simulink model "Motor_Cmd_varY"  (Simulink 7.9)
settings: Solver=FixedStepDiscrete  StartTime=0.0  StopTime=10  RelTol=1e-3  SampleTimeConstraint=STIndependent
PreLoadFcn:
  | Motor_Cmd_varY_selfinit
values from neighbouring files (symbols this model uses):
  lockDoor_cmdMotorVoltageValue = mpt.Parameter    [Motor_Cmd_varY_selfinit.m]
libraries: simulink x1
settings Model: RequirementInfo="{}  %GIDa_76f203d0_57c5_4172_aee2_9207869380ab"  Creator=fguerin  LastModifiedBy=klindqvi  CovMetricSettings=dc  CovHTMLOptions=-aTS=1 -bRG=1 -bTC=1 -hTR=0 -nFC=0 -scm=1 -bcm=1 -xEv=0  CovModelRefEnable=all
settings DataIOCC: ExternalInput=[t,u]  LimitDataPoints=off  SaveOutput=off  DSMLogging=off  SaveTime=off  SignalLoggingName=logsOut
settings OptimizationCC: InlineParams=on  InlineInvariantSignals=on  EnhancedBackFolding=on  ZeroExternalMemoryAtStartup=off  ZeroInternalMemoryAtStartup=off  EfficientFloat2IntCast=on  OptimizeModelRefInitCode=on  LifeSpan=1
settings DebuggingCC: ReadBeforeWriteMsg=EnableAllAsError  WriteAfterWriteMsg=EnableAllAsError  WriteAfterReadMsg=EnableAllAsError  AlgebraicLoopMsg=error  ArtificialAlgebraicLoopMsg=error  SaveWithDisabledLinksMsg=error  SaveWithParameterizedLinksMsg=error  CheckExecutionContextPreStartOutputMsg=on  CheckExecutionContextRuntimeOutputMsg=on  BlockPriorityViolationMsg=error  SolverPrmCheckMsg=none  MultiTaskCondExecSysMsg=warning  MultiTaskRateTransMsg=warning  IntegerOverflowMsg=none  ParameterUnderflowMsg=error  ParameterPrecisionLossMsg=error  ParameterTunabilityLossMsg=error  UnderSpecifiedDataTypeMsg=warning  UnnecessaryDatatypeConvMsg=warning  VectorMatrixConversionMsg=error  SignalLabelMismatchMsg=warning  SFcnCompatibilityMsg=error  BusObjectLabelMismatch=error  RootOutportRequireBusObject=error  AssertControl=DisableAll  ModelReferenceIOMsg=error  ModelReferenceIOMismatchMessage=error  ModelReferenceCSMismatchMessage=warning  UnknownTsInhSupMsg=error  ModelReferenceDataLoggingMessage=error  ModelReferenceSymbolNameMessage=none  StrictBusMsg=ErrorOnBusTreatedAsVector
settings HardwareCC: ProdLargestAtomicInteger=Long  ProdLargestAtomicFloat=Double  ProdIntDivRoundTo=Zero  ProdEndianess=BigEndian  ProdHWDeviceType=Freescale->MPC5500
settings SFSimCC: SimParseCustomCode=off
settings RTWCC: SystemTargetFile=ert.tlc  TemplateMakefile=ert_default_tmf  Description=Embedded Coder  GenerateReport=on  RTWVerbose=off  ProcessScript=ert_make_rtw_hook  IncludeHyperlinkInReport=on  GenerateTraceInfo=on  GenerateTraceReport=on  GenerateTraceReportSl=on  GenerateTraceReportSf=on  GenerateTraceReportEml=on  GenerateCodeMetricsReport=on
settings MATStruct: className=rtw.pil.Bullseye  argsAllComponents=[]  excludedModels=[]  includeReferencedModels=on  includeTopModel=on  enabled=off
settings CodeAppCC: ForceParamTrailComments=on  IgnoreCustomStorageClasses=off  IgnoreTestpoints=on  MangleLength=4  InlinedPrmAccess=Macros  ReqsInCode=on
settings ERTTargetCC: CodeReplacementLibrary=ANSI_C  MultiwordLength=2048  SupportAbsoluteTime=off  SupportNonFinite=off  SupportComplex=off  PortableWordSizes=on  InlinedParameterPlacement=NonHierarchical  ERTCustomFileTemplate=example_file_process.tlc  ConvertIfToSwitch=off  SuppressUnreachableDefaultCases=off
settings ConfigComp: Description=Design Verifier Custom Configuration Component  DVMaxProcessTime=600  DVDisplayUnsatisfiableObjectives=on  DVAutomaticStubbing=off  DVOutputDir=sldv_output  DVTestSuiteOptimization=CombinedObjectives  DVDataFileName=./Tests/$ModelName$_sldvdata  DVHarnessModelFileName=./Tests/$ModelName$_testHarness  DVModelReferenceHarness=on  DVSaveReport=on  DVReportFileName=ADL_Sim_SLDV.html

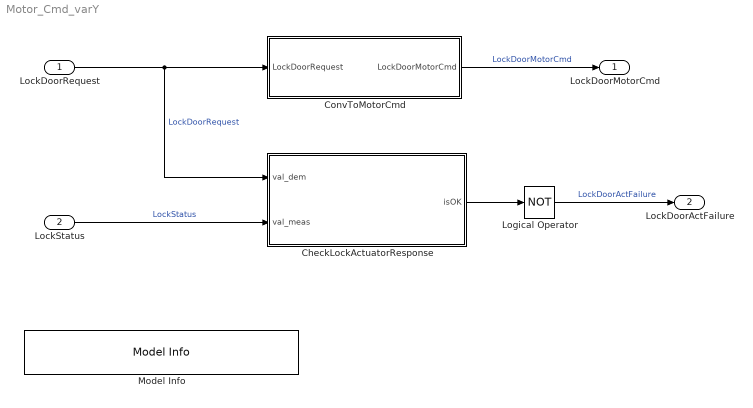
== system Motor_Cmd_varY ==
  LockDoorRequest : Inport  OutDataTypeStr=boolean  PortDimensions=1
  LockStatus : Inport  Port=2  OutDataTypeStr=Enum: ActuatorStatus  PortDimensions=1
  CheckLockActuatorResponse : MATLAB Function  RequirementInfo={'other' '..\doorlockingsystem_swr.doc' '@Simulink_requirement_item_3' 'true' 'REQ301 – A door lock failure should be reported if the door lock has not responded to command in 2 seconds.' '' } %GIDa_063ed5f7_a3e4_495a_bc51_85557e752733  TreatAsAtomicUnit=on
  ConvToMotorCmd : Subsystem
  Logical Operator : Logic  Operator=NOT  AllPortsSameDT=off  OutDataTypeStr=boolean
  Model Info : simulink/Model-Wide Utilities/Model Info  InitialBlockCM=RCS  BlockCM=RCS  Frame=on  DisplayStringWithTags=|  HorizontalTextAlignment=Center  LeftAlignmentValue=0.5  SourceBlockDiagram=Motor_Cmd_varY  TagMaxNumber=20  CMTag1=$Author: klindqvi $  CMTag2=$Date: 2012-03-27 11:02:37 +0100 (Tue, 27 Mar 2012) $  CMTag3=$Revision: 112 $  CMTag4=$Header: $  CMTag5=$Id: Motor_Cmd_varY.mdl 112 2012-03-27 10:02:37Z klindqvi $  CMTag6=$Locker: $  CMTag7=$RCSfile: $  CMTag8=$Source: $  CMTag9=$State: $
      | %<Author>
      | %<Revision>
      | %<Date>
  LockDoorMotorCmd : Outport  OutDataTypeStr=uint8  PortDimensions=1
  LockDoorActFailure : Outport  Port=2  OutDataTypeStr=boolean
  wires:
  CheckLockActuatorResponse/1(isOK) -> Logical Operator/1
  LockStatus/1 -> CheckLockActuatorResponse/2(val_meas)  "LockStatus"
  ConvToMotorCmd/1(LockDoorMotorCmd) -> LockDoorMotorCmd/1  "LockDoorMotorCmd"
  LockDoorRequest/1 -> CheckLockActuatorResponse/1(val_dem), ConvToMotorCmd/1(LockDoorRequest)  "LockDoorRequest"
  Logical Operator/1 -> LockDoorActFailure/1  "LockDoorActFailure"

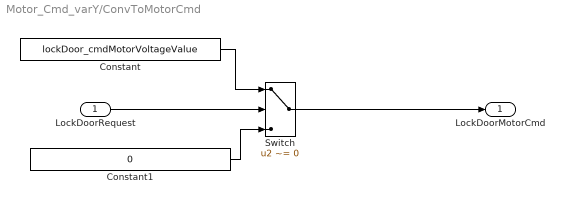
== system Motor_Cmd_varY/ConvToMotorCmd ==
  LockDoorRequest : Inport
  Constant : Constant  Value=lockDoor_cmdMotorVoltageValue  SampleTime=-1
  Constant1 : Constant  Value=0  OutDataTypeStr=Inherit: Inherit via back propagation  SampleTime=-1
  Switch : Switch  Criteria=u2 ~= 0  OutDataTypeStr=Inherit: Inherit via back propagation  InputSameDT=on
  LockDoorMotorCmd : Outport
  wires:
  Switch/1 -> LockDoorMotorCmd/1
  Constant1/1 -> Switch/3
  Constant/1 -> Switch/1
  LockDoorRequest/1 -> Switch/2

== matlab function CheckLockActuatorResponse ==
  settings: fimath=fimath('OverflowMode','wrap')
  data: val_dem input boolean size=1; isOK output boolean size=1; val_meas input Enum: ActuatorStatus size=1; lockDoor_responseTime parameter uint32 size=1
function isOK = VerifyResponseTime(val_dem, val_meas, lockDoor_responseTime)
%#eml
% This function checks that the feedback 
persistent last_demand
persistent sample_counter

% Initialize state variables
if isempty(last_demand)
    last_demand = val_dem;
end
if isempty(sample_counter)
    sample_counter = uint32(0);
end

%Initialize output
isOK = true;

% if demand has changed
if val_dem ~= last_demand
    % Update last demand and reset sample counter
    last_demand = val_dem;
    sample_counter =  uint32(0);
    isOK = true;
end

% If time to check measure value
if sample_counter >= lockDoor_responseTime
    if val_dem == true  && val_meas == ActuatorStatus.LOCK_POS || ...
       val_dem == false && val_meas == ActuatorStatus.UNLOCK_POS
        isOK = true;
    else
        % Error
        isOK = false;
    end
else    
    %Update sample counter
    sample_counter =  sample_counter + 1; 
end
